simulink model "state_feedback_controller_no_observer"  (R2018a)
settings: Solver=VariableStepAuto  StartTime=0.0  StopTime=10.0  RelTol=1e-3
undefined symbols (not defined in the file): K, sys, x0
settings Model: Creator=julio  LastModifiedBy=julio

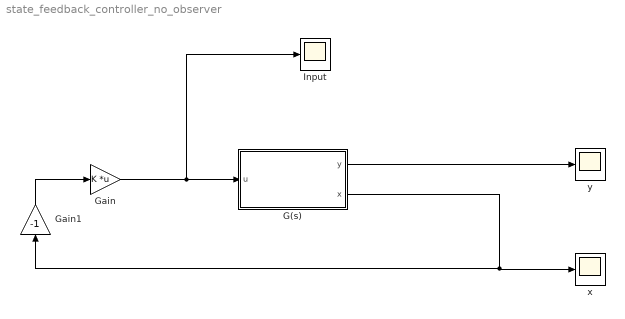
== system state_feedback_controller_no_observer ==
  G(s) : Subsystem
  Gain : Gain  Gain=K  Multiplication=Matrix(K*u)
  Gain1 : Gain  Gain=-1
  Input : Scope
  x : Scope
  y : Scope
  wires:
  G(s)/2(x) -> Gain1/1, x/1
  G(s)/1(y) -> y/1
  Gain/1 -> G(s)/1(u), Input/1
  Gain1/1 -> Gain/1

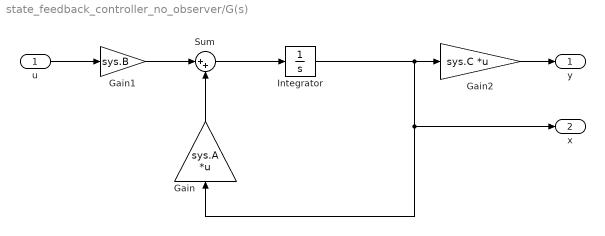
== system state_feedback_controller_no_observer/G(s) ==
  u : Inport
  Gain : Gain  Gain=sys.A  Multiplication=Matrix(K*u)
  Gain1 : Gain  Gain=sys.B
  Gain2 : Gain  Gain=sys.C  Multiplication=Matrix(K*u)
  Integrator : Integrator  InitialCondition=x0
  Sum : Sum  Inputs=|++
  y : Outport
  x : Outport  Port=2
  wires:
  u/1 -> Gain1/1
  Gain2/1 -> y/1
  Gain1/1 -> Sum/1
  Gain/1 -> Sum/2
  Sum/1 -> Integrator/1
  Integrator/1 -> x/1, Gain/1, Gain2/1
